simulink subsystem "KalmanFilter"  (R2021b)
settings: Solver=VariableStepAuto  StartTime=0.0  StopTime=10.0  RelTol=1e-3
settings Model: Creator=smryk  LastModifiedBy=lupas
settings DebuggingCC: UnconnectedInputMsg=none  UnconnectedOutputMsg=none  UnconnectedLineMsg=none
settings ModelReferenceCC: EnableRefExpFcnMdlSchedulingChecks=off
settings RTWCC: DLArmComputeVersion=20.02.1

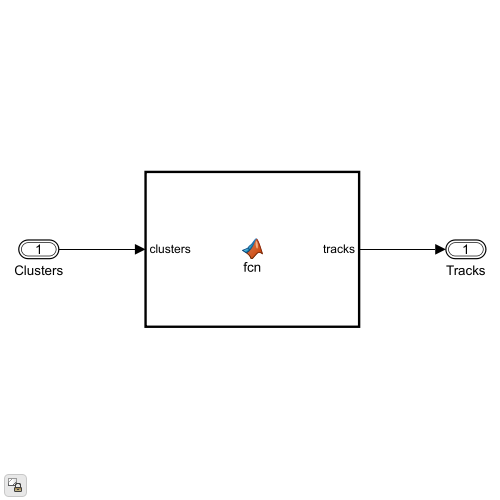
[thumbnail: Simulink's stored preview of the top-level diagram]
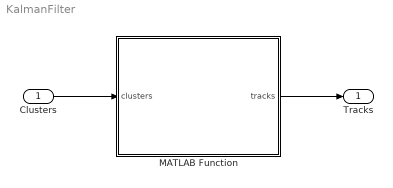
== system KalmanFilter ==
  Clusters : Inport  OutDataTypeStr=Bus: BusObjectDetections1
  MATLAB Function : MATLAB Function  TreatAsAtomicUnit=on
  Tracks : Outport  OutDataTypeStr=Bus: SystemTracks
  wires:
  Clusters/1 -> MATLAB Function/1(clusters)
  MATLAB Function/1(tracks) -> Tracks/1

== matlab function KalmanFilter/MATLAB Function ==
  data: clusters input Bus: BusObjectDetections1; tracks output Bus: SystemTracks
function tracks = fcn(clusters)

max_clust = 32


% EstimatesNext = zeros(6);
% EstimatesCurrent = zeros(6);
% UncertaintyNext = zeros(6, 6);
% UncertaintyCurrent = zeros(6, 6);
% KalmanGain = zeros(6, 6);
% ;
% intialEstimate = zeros(6, 1);
% initialUncertainty = diag([500 500 500 500 500 500]);

dt = 1;
StDev = 0.2;
MeasureError = 3;

ZeroMat = zeros(3);
A = [1 dt (0.5*dt^2)
     0 1  dt
     0 0  1];
F = [A ZeroMat
     ZeroMat A];

B = [dt^2/4 dt^3/2 dt^2/2
     dt^3/2 dt^2   dt
     dt^2/2 dt     1];

Q = [B ZeroMat
     ZeroMat B] * StDev^2;

R = [MeasureError^2 0
     0 MeasureError^2];

C = [1 0 0];
D = [0 1 0];
E = [0 0 0];
H = [C E
     E C
     E E
     D E
     E D
     E E];



% EstimatesNext = F*intialEstimate;
% UncertaintyNext = F*initialUncertainty*transpose(F)+Q;

for i = 1:
KalmanGain =  (UncertaintyNext*transpose(H)) / (H*UncertaintyNext * transpose(H) + R);
EstimatesCurrent = EstimatesNext + KalmanGain * ([xMeasured(1); yMeasured(1)] - H*EstimatesNext);

identminus = eye(6) - KalmanGain * H;
UncertaintyCurrent = identminus * UncertaintyNext * transpose(identminus) + KalmanGain*R*transpose(KalmanGain);


EstimatesNext = F*EstimatesCurrent;
UncertaintyNext = F * UncertaintyCurrent * transpose(F) + Q;

%EstimatesCurrent(1,:)
%plot(xExact, yExact,'b', xMeasured, yMeasured, '.g', EstimatesCurrent, EstimatesCurrent, '.r');
%legend('Exact', 'Measured', 'Estimates'); % legend

% 
% placeHolderAttributes.TargetIndex = 1;
% placeHolderAttributes.SNR = 1;
% 
% tracks.NumTracks = 0;
% 
% fakeTrack.TrackID = uint32(1);
% fakeTrack.BranchID = uint32(1);
% fakeTrack.SourceIndex = uint32(1);
% fakeTrack.UpdateTime = 0.1;
% fakeTrack.Age = uint32(1);
% fakeTrack.State = [0; 0; 0; 0; 0; 0];
% fakeTrack.StateCovariance = zeros(6,6);
% fakeTrack.ObjectClassID = 1;
% fakeTrack.TrackLogic = trackLogicType.History;
% fakeTrack.TrackLogicState = [true true true];
% fakeTrack.IsConfirmed = boolean(0);
% fakeTrack.IsCoasted = boolean(false);
% fakeTrack.IsSelfReported = boolean(false);
% fakeTrack.ObjectAttributes = [placeHolderAttributes; placeHolderAttributes];
